simulink model "acrobot2"  (R2017a)
settings: Solver=ode2  StartTime=0.0  StopTime=2  FixedStep=.1  RelTol=1e-3
values from neighbouring files (symbols this model uses):
  g = 9.8    [acrobot_m.m]
  Kd1 = 0    [acrobot_m.m]
  Kd2 = 00    (= 0)    [acrobot_m.m]
  Ki1 = 0    [acrobot_m.m]
  Ki2 = 0    [acrobot_m.m]
  Kp1 = 0    [acrobot_m.m]
  Kp2 = 00    (= 0)    [acrobot_m.m]
  l1 = 1    [acrobot_m.m]
  l2 = 1    [acrobot_m.m]
  m1 = 1    [acrobot_m.m]
  m2 = 1    [acrobot_m.m]
settings Model: Creator=SHREYASH  LastModifiedBy=SHREYASH
settings SolverCC: AlgebraicLoopSolver=LineSearch

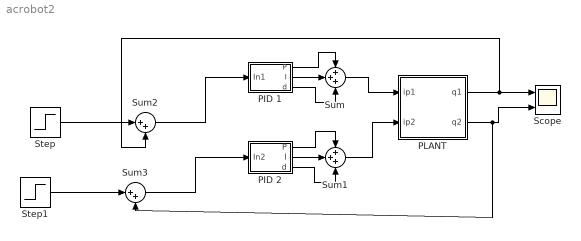
== system acrobot2 ==
  PID 1 : Subsystem
  PID 2 : Subsystem
  PLANT : Subsystem
  Scope : Scope  NumInputPorts=2
  Step : Step  Time=pi  SampleTime=0  VectorParams1D=off
  Step1 : Step  Time=0  SampleTime=0  VectorParams1D=off
  Sum : Sum  Inputs=3
  Sum1 : Sum  Inputs=3
  Sum2 : Sum  Inputs=|++
  Sum3 : Sum  Inputs=|++
  wires:
  Sum/1 -> PLANT/1("ip1 ")
  PID 1/1(P) -> Sum/1
  PID 1/2(I) -> Sum/2
  PID 1/3(d) -> Sum/3
  PID 2/3(d) -> Sum1/3
  PID 2/2(I) -> Sum1/2
  PID 2/1(P) -> Sum1/1
  Sum1/1 -> PLANT/2(ip2)
  Sum2/1 -> PID 1/1("In1 ")
  PLANT/2(q2) -> Sum3/2, Scope/2
  Step/1 -> Sum2/1
  PLANT/1("q1 ") -> Sum2/2, Scope/1
  Step1/1 -> Sum3/1
  Sum3/1 -> PID 2/1("In2 ")

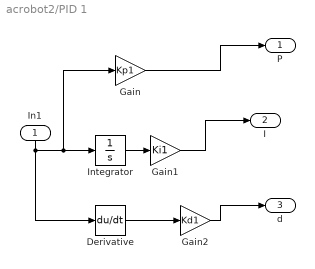
== system acrobot2/PID 1 ==
  "In1 " : Inport
  Derivative : Derivative  CoefficientInTFapproximation=0
  Gain : Gain  Gain=Kp1
  Gain1 : Gain  Gain=Ki1
  Gain2 : Gain  Gain=Kd1
  Integrator : Integrator
  P : Outport
  I : Outport  Port=2
  d : Outport  Port=3
  wires:
  Gain2/1 -> d/1
  Gain/1 -> P/1
  Integrator/1 -> Gain1/1
  Derivative/1 -> Gain2/1
  "In1 "/1 -> Gain/1, Integrator/1, Derivative/1
  Gain1/1 -> I/1

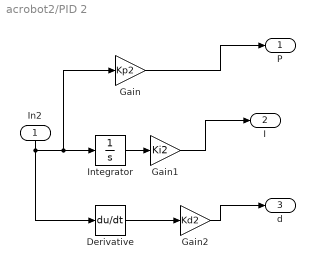
== system acrobot2/PID 2 ==
  "In2 " : Inport
  Derivative : Derivative  CoefficientInTFapproximation=0
  Gain : Gain  Gain=Kp2
  Gain1 : Gain  Gain=Ki2
  Gain2 : Gain  Gain=Kd2
  Integrator : Integrator
  P : Outport
  I : Outport  Port=2
  d : Outport  Port=3
  wires:
  Gain1/1 -> I/1
  "In2 "/1 -> Derivative/1, Integrator/1, Gain/1
  Derivative/1 -> Gain2/1
  Integrator/1 -> Gain1/1
  Gain/1 -> P/1
  Gain2/1 -> d/1

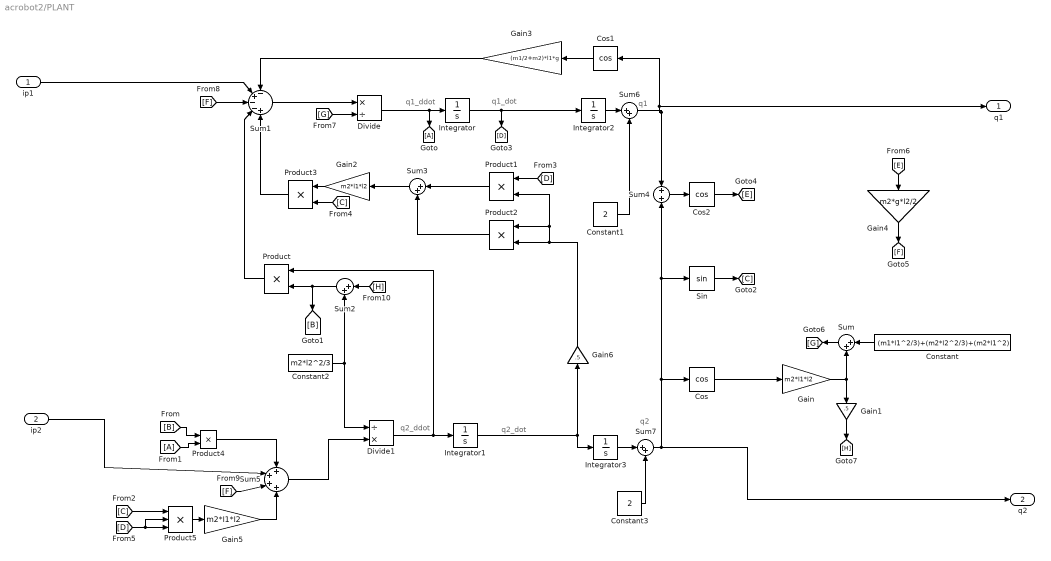
== system acrobot2/PLANT ==
  note: q2
  note: q1
  note: q2_dot
  note: q1_dot
  note: q2_ddot
  note: q1_ddot
  "ip1 " : Inport
  ip2 : Inport  Port=2
  Constant : Constant  Value=(m1*l1^2/3)+(m2*l2^2/3)+(m2*l1^2)
  Constant1 : Constant  Value=2
  Constant2 : Constant  Value=m2*l2^2/3
  Constant3 : Constant  Value=2
  Cos : Trigonometry  Operator=cos
  Cos1 : Trigonometry  Operator=cos
  Cos2 : Trigonometry  Operator=cos
  Divide : Product  Inputs=*/
  Divide1 : Product  Inputs=/*
  Gain : Gain  Gain=m2*l1*l2
  Gain1 : Gain  Gain=.5
  Gain2 : Gain  Gain=m2*l1*l2
  Gain3 : Gain  Gain=(m1/2+m2)*l1*g
  Gain4 : Gain  Gain=m2*g*l2/2
  Gain5 : Gain  Gain=m2*l1*l2
  Gain6 : Gain  Gain=.5
  Integrator{,1..3} (4 alike) : Integrator
  Product{,1..4} (5 alike) : Product
  Product5 : Product  Inputs=3
  Sin : Trigonometry
  Sum{,2..3,6..7} (5 alike) : Sum  Inputs=|++
  Sum1 : Sum  Inputs=-+--+
  Sum4 : Sum  Inputs=2
  Sum5 : Sum  Inputs=++++
  "q1 " : Outport
  q2 : Outport  Port=2
  wires:
  Gain1/1 -> [H]
  [F] -> Sum5/3
  [G] -> Divide/2
  Sum/1 -> [G]
  [H] -> Sum2/1
  [E] -> Gain4/1
  [F] -> Sum1/3
  Cos2/1 -> [E]
  Sin/1 -> [C]
  Divide/1 -> Integrator/1, [A]
  Sum1/1 -> Divide/1
  Sum3/1 -> Gain2/1
  Cos/1 -> Gain/1
  Gain2/1 -> Product3/1
  Gain4/1 -> [F]
  Cos1/1 -> Gain3/1
  Divide1/1 -> Product/1, Integrator1/1
  Sum5/1 -> Divide1/2
  Product3/1 -> Sum1/5
  Product/1 -> Sum1/4
  [A] -> Product4/2
  Sum4/1 -> Cos2/1
  Product2/1 -> Sum3/2
  [B] -> Product4/1
  Constant2/1 -> Divide1/1, Sum2/2
  Gain3/1 -> Sum1/1
  Product4/1 -> Sum5/1
  Constant/1 -> Sum/1
  Sum2/1 -> [B], Product/2
  Product1/1 -> Sum3/1
  Integrator/1 -> [D], Integrator2/1
  Integrator1/1 -> Integrator3/1, Gain6/1
  Product5/1 -> Gain5/1
  [C] -> Product3/2
  [D] -> Product5/2, Product5/3
  [C] -> Product5/1
  [D] -> Product1/1
  Gain5/1 -> Sum5/4
  "ip1 "/1 -> Sum1/2
  Gain/1 -> Gain1/1, Sum/2
  Gain6/1 -> Product1/2, Product2/1, Product2/2
  ip2/1 -> Sum5/2
  Constant1/1 -> Sum6/2
  Integrator2/1 -> Sum6/1
  Sum6/1 -> "q1 "/1, Cos1/1, Sum4/1
  Integrator3/1 -> Sum7/1
  Sum7/1 -> q2/1, Cos/1, Sin/1, Sum4/2
  Constant3/1 -> Sum7/2
